simulink library "read"  (R2024a)
settings: Solver=VariableStepAuto  StartTime=0.0  StopTime=10.0  RelTol=1e-3
settings Model: Creator=eikel  LastModifiedBy=adriaeik

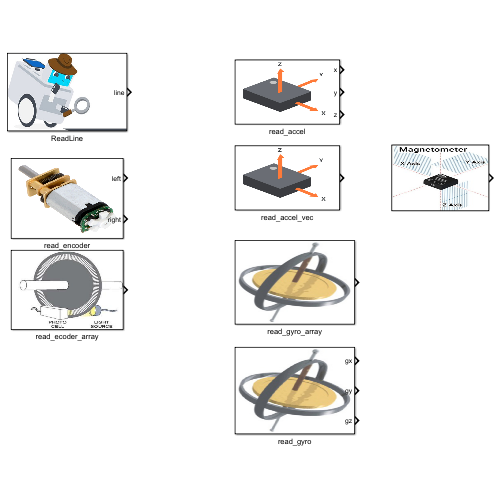
[thumbnail: Simulink's stored preview of the top-level diagram]
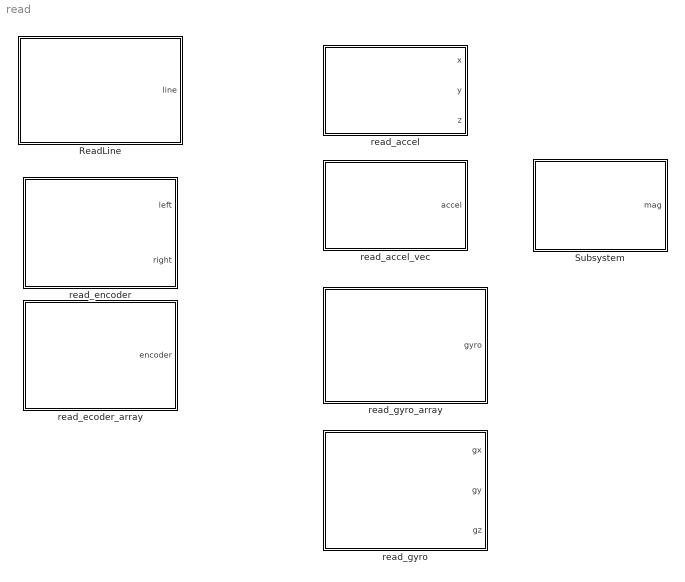
== system read ==
  ReadLine : Subsystem
      mask Display: image('lineDetector.jpg');
  Subsystem : Subsystem
      mask Display: image('mag.jpg');
  read_accel : Subsystem
      mask Display: image('accel.png');
  read_accel_vec : Subsystem
      mask Display: image('accel.png');
  read_ecoder_array : Subsystem
      mask Display: image('encoder_light.png');
  read_encoder : Subsystem
      mask Display: image('encoder_pololu.jpg');
  read_gyro : Subsystem
      mask Display: image('Gyroscope.jpg');
  read_gyro_array : Subsystem
      mask Display: image('Gyroscope.jpg');

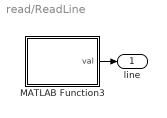
== system read/ReadLine ==
  MATLAB Function3 : MATLAB Function  TreatAsAtomicUnit=on
  line : Outport
  wires:
  MATLAB Function3/1(val) -> line/1

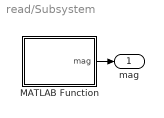
== system read/Subsystem ==
  MATLAB Function : MATLAB Function  TreatAsAtomicUnit=on
  mag : Outport
  wires:
  MATLAB Function/1(mag) -> mag/1

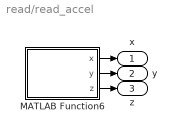
== system read/read_accel ==
  MATLAB Function6 : MATLAB Function  TreatAsAtomicUnit=on
  x : Outport
  y : Outport  Port=2
  z : Outport  Port=3
  wires:
  MATLAB Function6/3(z) -> z/1
  MATLAB Function6/1(x) -> x/1
  MATLAB Function6/2(y) -> y/1

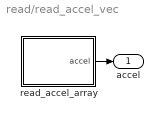
== system read/read_accel_vec ==
  read_accel_array : MATLAB Function  TreatAsAtomicUnit=on
  accel : Outport
  wires:
  read_accel_array/1(accel) -> accel/1

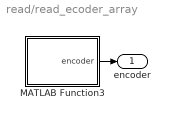
== system read/read_ecoder_array ==
  MATLAB Function3 : MATLAB Function  TreatAsAtomicUnit=on
  encoder : Outport
  wires:
  MATLAB Function3/1(encoder) -> encoder/1

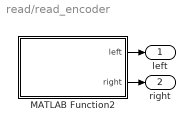
== system read/read_encoder ==
  MATLAB Function2 : MATLAB Function  TreatAsAtomicUnit=on
  left : Outport
  right : Outport  Port=2
  wires:
  MATLAB Function2/2(right) -> right/1
  MATLAB Function2/1(left) -> left/1

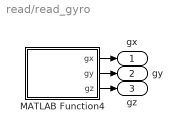
== system read/read_gyro ==
  MATLAB Function4 : MATLAB Function  TreatAsAtomicUnit=on
  gx : Outport
  gy : Outport  Port=2
  gz : Outport  Port=3
  wires:
  MATLAB Function4/1(gx) -> gx/1
  MATLAB Function4/2(gy) -> gy/1
  MATLAB Function4/3(gz) -> gz/1

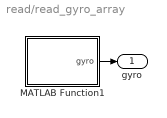
== system read/read_gyro_array ==
  MATLAB Function1 : MATLAB Function  TreatAsAtomicUnit=on
  gyro : Outport
  wires:
  MATLAB Function1/1(gyro) -> gyro/1

== matlab function read/Subsystem/MATLAB Function ==
  data: mag output
function mag = read_mag()
    coder.extrinsic('get_mag');
    [x, y, z] = get_mag();
    mag = [0 0 0];
    if ~isnan(x), mag(1) = x; end
    if ~isnan(y), mag(2) = y; end
    if ~isnan(z), mag(3) = z; end
end

== matlab function read/read_encoder/MATLAB Function2 ==
  data: left output; right output
function [left, right] = read_encoder()
    coder.extrinsic('get_encoder');
    [l_tmp, r_tmp] = get_encoder();

    left  = 0;
    right = 0;

    if ~isnan(l_tmp),  left  = l_tmp;  end
    if ~isnan(r_tmp),  right = r_tmp;  end
end

== matlab function read/ReadLine/MATLAB Function3 ==
  data: val output
function val = read_line()
    coder.extrinsic('get_line');  % Kallar på ekstern .m-fil
    val = 0;                      % Initier til 0
    tmp = get_line();            % Hent verdi

    if ~isnan(tmp)
        val = tmp;
    end
end

== matlab function read/read_ecoder_array/MATLAB Function3 ==
  data: encoder output
function encoder = read_encoder()
    coder.extrinsic('get_encoder');
    [l, r] = get_encoder();
    encoder = [0 0];
    if ~isnan(l), encoder(1) = l; end
    if ~isnan(r), encoder(2) = r; end
end

== matlab function read/read_gyro/MATLAB Function4 ==
  data: gx output; gy output; gz output
function [gx, gy, gz] = read_gyro()
    coder.extrinsic('get_gyro');
    [gx_tmp, gy_tmp, gz_tmp] = get_gyro();

    gx = 0; if ~isnan(gx_tmp), gx = gx_tmp; end
    gy = 0; if ~isnan(gy_tmp), gy = gy_tmp; end
    gz = 0; if ~isnan(gz_tmp), gz = gz_tmp; end
end

== matlab function read/read_accel_vec/read_accel_array ==
  data: accel output
function accel = read_accel()
    coder.extrinsic('get_accel');
    [x, y, z] = get_accel();
    accel = [0 0 0];
    if ~isnan(x), accel(1) = x; end
    if ~isnan(y), accel(2) = y; end
    if ~isnan(z), accel(3) = z; end
end

== matlab function read/read_accel/MATLAB Function6 ==
  data: x output; y output; z output
function [x, y, z] = read_accel()
    coder.extrinsic('get_accel');
    [x_tmp, y_tmp, z_tmp] = get_accel();

    x = 0; if ~isnan(x_tmp), x = x_tmp; end
    y = 0; if ~isnan(y_tmp), y = y_tmp; end
    z = 0; if ~isnan(z_tmp), z = z_tmp; end
end

== matlab function read/read_gyro_array/MATLAB Function1 ==
  data: gyro output
function gyro = read_gyro_vec()
    coder.extrinsic('get_gyro');
    [x, y, z] = get_gyro();
    gyro = [0 0 0];
    if ~isnan(x), gyro(1) = x; end
    if ~isnan(y), gyro(2) = y; end
    if ~isnan(z), gyro(3) = z; end
end
